simulink model "sim3"  (R2022b)
settings: Solver=VariableStepAuto  StartTime=0.0  StopTime=0.1  MaxStep=1e-6  RelTol=1e-3
values from neighbouring files (symbols this model uses):
  J = 3.6e-4    (= 0.00036)    [setup.m]
  ke = 0.5    [setup.m]
  km = 0.5    [setup.m]
  L = 1e-3    (= 0.001)    [setup.m]
  R = 0.22    [setup.m]
settings Model: Creator=serez  LastModifiedBy=serez

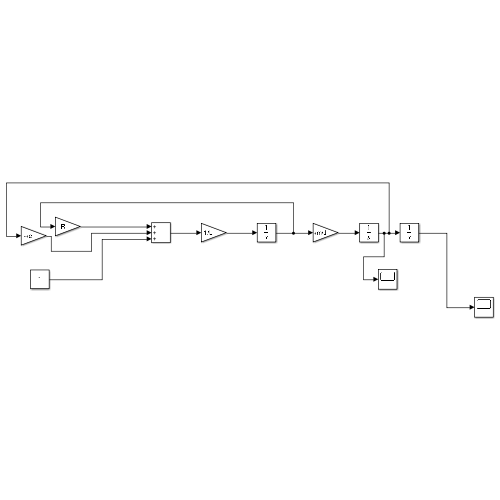
[thumbnail: Simulink's stored preview of the top-level diagram]
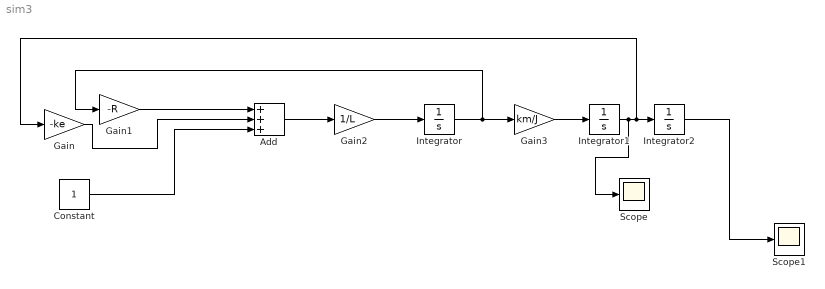
== system sim3 ==
  Add : Sum  Inputs=+++
  Constant : Constant
  Gain : Gain  Gain=-ke
  Gain1 : Gain  Gain=-R
  Gain2 : Gain  Gain=1/L
  Gain3 : Gain  Gain=km/J
  Integrator : Integrator
  Integrator1 : Integrator
  Integrator2 : Integrator
  Scope : Scope
  Scope1 : Scope
  wires:
  Gain1/1 -> Add/1
  Constant/1 -> Add/3
  Gain/1 -> Add/2
  Add/1 -> Gain2/1
  Gain2/1 -> Integrator/1
  Integrator/1 -> Gain1/1, Gain3/1
  Integrator1/1 -> Scope/1, Gain/1, Integrator2/1
  Gain3/1 -> Integrator1/1
  Integrator2/1 -> Scope1/1
